simulink model "First_1"  (R2015b)
settings: Solver=FixedStepAuto  StartTime=0.0  StopTime=inf  FixedStep=0.00000001  RelTol=1e-3
settings Model: Creator=User  LastModifiedBy=User

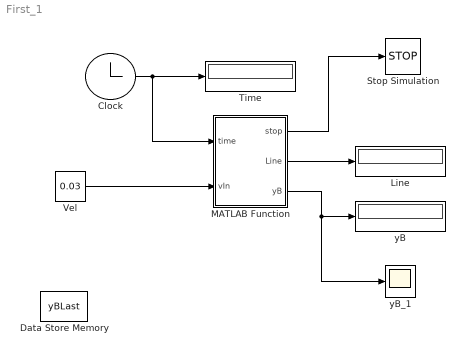
== system First_1 ==
  Clock : Clock
  Data Store Memory : DataStoreMemory  DataStoreName=yBLast  ReadBeforeWriteMsg=warning  WriteAfterWriteMsg=warning  WriteAfterReadMsg=warning  OutDataTypeStr=double
  Line : Display
  MATLAB Function : MATLAB Function  TreatAsAtomicUnit=on
  Stop Simulation : Stop
  Time : Display
  Vel : Constant  Value=0.03
  yB : Display
  yB_1 : Scope
  wires:
  Clock/1 -> MATLAB Function/1(time), Time/1
  Vel/1 -> MATLAB Function/2(vIn)
  MATLAB Function/1(stop) -> Stop Simulation/1
  MATLAB Function/2(Line) -> Line/1
  MATLAB Function/3(yB) -> yB_1/1, yB/1

== matlab function First_1/MATLAB Function ==
  data: time input; stop output; vIn input; Line output; yB output; yBLast data_store_memory
function [stop,Line,yB] = fcn(time,vIn)
%#codegen

global yBLast;
%persistent yBL;
Line = vIn*time;
if (Line >= 0.1)
    stop = 1;
else
    stop = 0;
end

m = 0.000221;
pi = 3.1415926535;
alfaG = 45;
gammaG = 90-alfaG;
gammaR = (gammaG*pi)/180;
E = 2*(10^11);
d = 0.001;
dIn = 0.0008;
s = pi*(d/2)*(d/2)*Line;
rho = 1300;

%needleF =  0.5; 
cF  = 1.15;%0.82;%(2*(needleF))/(rho*vIn*vIn*s);

envF   = cF*s*( (rho*vIn*vIn)/2  );  
envFp  = envF*cos(gammaR);
iIx    = ((Line)*((d^3) - (dIn^3)))/12;
if iIx == 0
    yB = 0;
else
yB     =  yBLast + 1000*(envFp*((Line)^3))/(3*E*iIx);
yBLast = yB;
end
end
